simulink model "SIM"  (R2022b)
settings: Solver=VariableStepAuto  StartTime=0.0  StopTime=800  FixedStep=CONTROL_CONST.dt  MaxStep=0.05  RelTol=1e-3
settings Model: Creator=19114  LastModifiedBy=19114

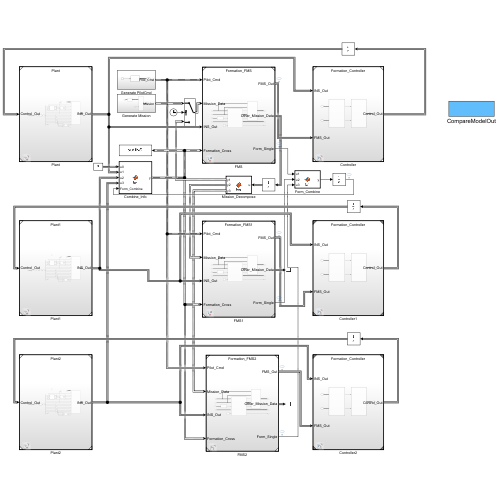
[thumbnail: Simulink's stored preview of the top-level diagram]
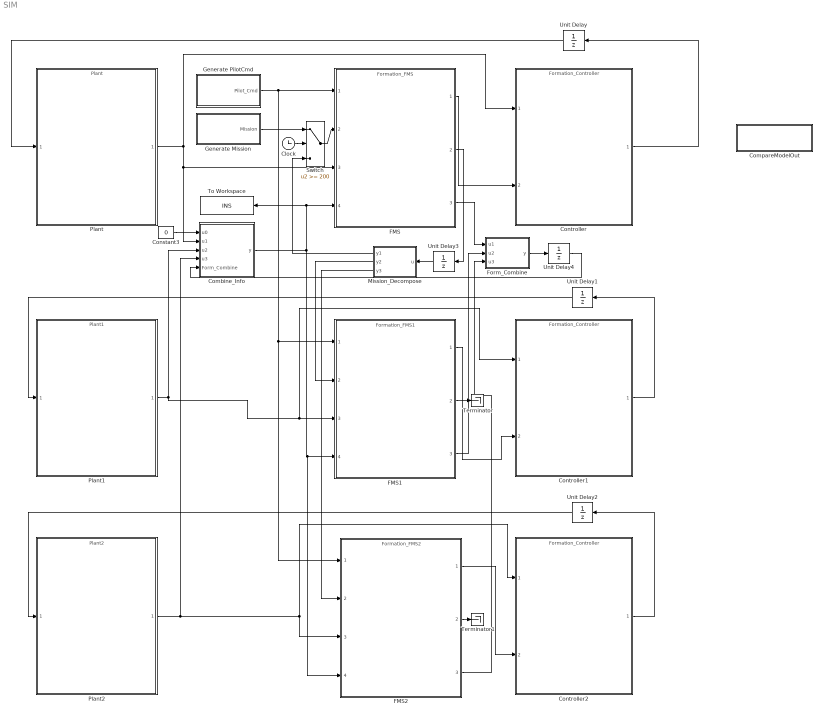
== system SIM ==
  Clock : Clock
  Combine_Info : MATLAB Function  TreatAsAtomicUnit=on
  CompareModelOut : Subsystem
      settings: OpenFcn=compareModelOut;
  Constant3 : Constant  Value=0  OutDataTypeStr=Bus: Formation_Cross_Bus
  Controller : ModelReference  ModelNameDialog=Formation_Controller.slx  SimulationMode=Normal  ModelReferenceVersion=1.315
  Controller1 : ModelReference  ModelNameDialog=Formation_Controller.slx  SimulationMode=Normal  ModelReferenceVersion=1.315
  Controller2 : ModelReference  ModelNameDialog=Formation_Controller.slx  SimulationMode=Normal  ModelReferenceVersion=1.315
  FMS : ModelReference  ModelNameDialog=Formation_FMS.slx  SimulationMode=Normal  ModelReferenceVersion=1.159
  FMS1 : ModelReference  ModelNameDialog=Formation_FMS1.slx  SimulationMode=Normal  ModelReferenceVersion=1.132
  FMS2 : ModelReference  ModelNameDialog=Formation_FMS2.slx  SimulationMode=Normal  ModelReferenceVersion=1.132
  Form_Combine : MATLAB Function  TreatAsAtomicUnit=on
  Generate Mission : Subsystem
  Generate PilotCmd : Subsystem
  Mission_Decompose : MATLAB Function  TreatAsAtomicUnit=on
  Plant : ModelReference  ModelNameDialog=Plant.slx  SimulationMode=Normal  ModelReferenceVersion=1.90
  Plant1 : ModelReference  ModelNameDialog=Plant1.slx  SimulationMode=Normal  ModelReferenceVersion=1.83
  Plant2 : ModelReference  ModelNameDialog=Plant2.slx  SimulationMode=Normal  ModelReferenceVersion=1.83
  Switch : Switch  Threshold=200  SaturateOnIntegerOverflow=off  InputSameDT=off
  Terminator : Terminator
  Terminator1 : Terminator
  To Workspace : ToWorkspace  VariableName=INS  SaveFormat=Timeseries  SampleTime=-1
  Unit Delay{,1..4} (5 alike) : UnitDelay  SampleTime=-1  HasFrameUpgradeWarning=on
  wires:
  Controller/1 -> Unit Delay/1
  Unit Delay/1 -> Plant/1
  Constant3/1 -> Combine_Info/1(u0)
  Plant/1 -> FMS/3, Combine_Info/2(u1), Controller/1
  Combine_Info/1(y) -> FMS/4, To Workspace/1, FMS2/4, FMS1/4
  Mission_Decompose/1(y1) -> Switch/3
  FMS/1 -> Controller/2
  Generate PilotCmd/1(Pilot_Cmd) -> FMS2/1, FMS1/1, FMS/1
  Controller1/1 -> Unit Delay1/1
  Controller2/1 -> Unit Delay2/1
  FMS1/1 -> Controller1/2
  FMS2/1 -> Controller2/2
  FMS1/2 -> Terminator/1
  FMS2/2 -> Terminator1/1
  Plant2/1 -> Combine_Info/4(u3), FMS2/3, Controller2/1
  Plant1/1 -> FMS1/3, Controller1/1, Combine_Info/3(u2)
  FMS/2 -> Unit Delay3/1
  Mission_Decompose/2(y2) -> FMS1/2
  Unit Delay1/1 -> Plant1/1
  Mission_Decompose/3(y3) -> FMS2/2
  Unit Delay3/1 -> Mission_Decompose/1(u)
  Generate Mission/1(Mission) -> Switch/1
  Switch/1 -> FMS/2
  Clock/1 -> Switch/2
  FMS/3 -> Form_Combine/1(u1)
  FMS1/3 -> Form_Combine/2(u2)
  FMS2/3 -> Form_Combine/3(u3)
  Unit Delay4/1 -> Combine_Info/5(Form_Combine)
  Form_Combine/1(y) -> Unit Delay4/1
  Unit Delay2/1 -> Plant2/1

== system SIM/CompareModelOut ==

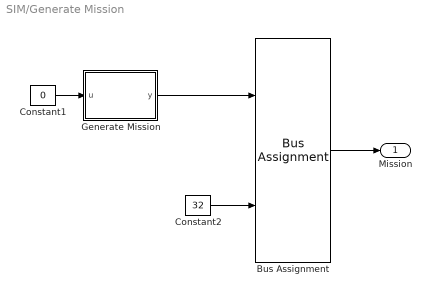
== system SIM/Generate Mission ==
  Bus Assignment : BusAssignment  AssignedSignals=timestamp
  Constant1 : Constant  Value=0  OutDataTypeStr=Bus: Mission_Data_Bus
  Constant2 : Constant  Value=32  OutDataTypeStr=uint32
  Generate Mission : MATLAB Function  TreatAsAtomicUnit=on
  Mission : Outport
  wires:
  Generate Mission/1(y) -> Bus Assignment/1
  Constant1/1 -> Generate Mission/1(u)
  Bus Assignment/1 -> Mission/1
  Constant2/1 -> Bus Assignment/2

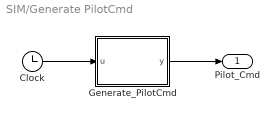
== system SIM/Generate PilotCmd ==
  Clock : Clock
  Generate_PilotCmd : MATLAB Function  TreatAsAtomicUnit=on
  Pilot_Cmd : Outport
  wires:
  Clock/1 -> Generate_PilotCmd/1(u)
  Generate_PilotCmd/1(y) -> Pilot_Cmd/1

== matlab function SIM/Generate PilotCmd/Generate_PilotCmd ==
  data: u input; y output Bus: Pilot_Cmd_Bus
function y = fcn(u)

if u < 0
    y.timestamp = uint32(0);
    y.mode = uint32(PilotMode.None);
elseif u < 100
    y.timestamp = uint32(1);
    y.mode = uint32(PilotMode.FormAssemble); % FormAssemble
else
    y.timestamp = uint32(1);
    y.mode = uint32(PilotMode.FormAssemble);
end

== matlab function SIM/Generate Mission/Generate Mission ==
  data: y output Bus: Mission_Data_Bus; u input Bus: Mission_Data_Bus
 function y  = fcn(u)

u.timestamp   = uint32(0);
u.type = uint32(3);
u.valid_items = uint8(4);

u.x(1) = single(4000);
u.y(1) = single(4000);
u.z(1) = single(1000);

u.x(2) = single(8000);
u.y(2) = single(4000);
u.z(2) = single(1000);

u.x(3) = single(8000);
u.y(3) = single(1000);
u.z(3) = single(1000);

u.x(4) = single(4000);
u.y(4) = single(1000);
u.z(4) = single(1000);


y = u;

== matlab function SIM/Mission_Decompose ==
  data: u input Bus: Other_Mission_Data_Bus; y1 output Bus: Mission_Data_Bus; y2 output Bus: Mission_Data_Bus; y3 output Bus: Mission_Data_Bus
function [y1,y2,y3] = fcn(u)

y1.timestamp = u.timestamp;
y1.type = u.type(1);
y1.valid_items = u.valid_items(1);
y1.x = u.x(1, :)';
y1.y = u.y(1, :)';
y1.z = u.z(1, :)';
y1.heading = u.heading(1, :)';
y1.ext1 = u.ext1(1, :)';
y1.ext2 = u.ext2(1, :)';

y2.timestamp = u.timestamp;
y2.type = u.type(2);
y2.valid_items = u.valid_items(2);
y2.x = u.x(2, :)';
y2.y = u.y(2, :)';
y2.z = u.z(2, :)';
y2.heading = u.heading(2, :)';
y2.ext1 = u.ext1(2, :)';
y2.ext2 = u.ext2(2, :)';

y3.timestamp = u.timestamp;
y3.type = u.type(3);
y3.valid_items = u.valid_items(3);
y3.x = u.x(3, :)';
y3.y = u.y(3, :)';
y3.z = u.z(3, :)';
y3.heading = u.heading(3, :)';
y3.ext1 = u.ext1(3, :)';
y3.ext2 = u.ext2(3, :)';

== matlab function SIM/Combine_Info ==
  settings: updateMethod=DISCRETE
  data: u0 input; y output Bus: Formation_Cross_Bus; u1 input; u2 input; u3 input; Form_Combine input
function y = fcn(u0, u1, u2, u3, Form_Combine)

persistent out;

if isempty(out)
    out = u0;
end

out.x_R(1) = u1.x_R;
out.x_R(2) = u2.x_R;
out.x_R(3) = u3.x_R;

out.y_R(1) = u1.y_R;
out.y_R(2) = u2.y_R;
out.y_R(3) = u3.y_R;

out.h_R(1) = u1.h_R;
out.h_R(2) = u2.h_R;
out.h_R(3) = u3.h_R;

out.vn(1) = u1.vn;
out.vn(2) = u2.vn;
out.vn(3) = u3.vn;

out.ve(1) = u1.ve;
out.ve(2) = u2.ve;
out.ve(3) = u3.ve;

out.vd(1) = u1.vd;
out.vd(2) = u2.vd;
out.vd(3) = u3.vd;

out.left_time(1) = Form_Combine(1);
out.left_time(2) = Form_Combine(2);
out.left_time(3) = Form_Combine(3);

y = out;

== matlab function SIM/Form_Combine ==
  data: u1 input; y output; u2 input; u3 input
function y = fcn(u1, u2, u3)

y = [u1 u2 u3];
